simulink model "proj_2"  (R2013a)
settings: Solver=ode45  StartTime=0.0  StopTime=15  RelTol=1e-3
settings Model: Creator=sivom  LastModifiedBy=sivom
settings DataIOCC: SignalLoggingSaveFormat=ModelDataLogs
settings DebuggingCC: SolverPrmCheckMsg=none  MultiTaskDSMMsg=warning  MultiTaskCondExecSysMsg=none  StrictBusMsg=None
settings RTWCC: IncludeERTFirstTime=on
settings GRTTargetCC: CodeReplacementLibrary=None  CPPClassGenCompliant=on

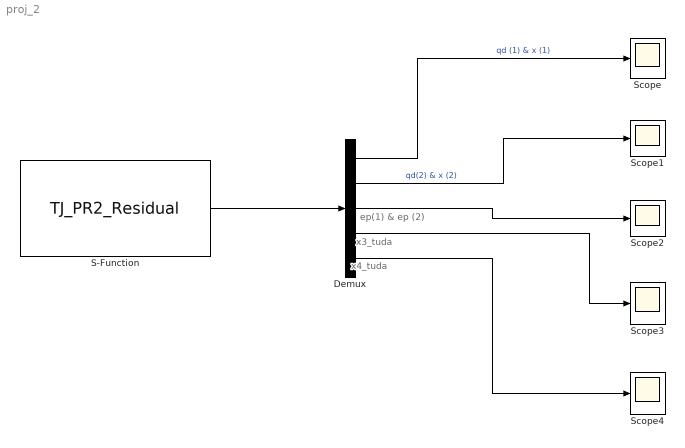
== system proj_2 ==
  note: x4_tuda
  note: x3_tuda
  note: ep(1) & ep (2)
  Demux : Demux  Outputs=5
  S-Function : S-Function  FunctionName=TJ_PR2_Residual  EnableBusSupport=off
  Scope{,1..4} (5 alike) : Scope
      Scope settings: ShowLegends=on
      Scope2 settings: SaveName=ScopeData2
      Scope3 settings: SaveName=ScopeData3
      Scope4 settings: SaveName=ScopeData4
  wires:
  Demux/1 -> Scope/1  "qd (1) & x (1)"
  Demux/2 -> Scope1/1  "qd(2) & x (2)"
  Demux/3 -> Scope2/1
  Demux/4 -> Scope3/1
  S-Function/1 -> Demux/1
  Demux/5 -> Scope4/1
